simulink model "EMplanner_cs2018a"  (R2018a)
settings: Solver=ode5  StartTime=0.0  StopTime=50  FixedStep=1/1000  RelTol=1e-3
PreLoadFcn:
  | mbxruntime.callbacks.PreLoadFcn(bdroot);
PostLoadFcn:
  | mbxruntime.callbacks.PostLoadFcn(bdroot);
InitFcn:
  | mbxruntime.callbacks.InitFcn(bdroot);
StartFcn:
  | mbxruntime.callbacks.StartFcn(bdroot);
StopFcn:
  | mbxruntime.callbacks.StopFcn(bdroot);
model workspace (MAT data in the model file):
  mbox_table : struct (value not decoded)
  model_closed = 0
  sim_status = 0
values from neighbouring files (symbols this model uses):
  c_factor = 43.75    [emplanner_init.m]
  cf = -175016    [emplanner_init.m]
  cr = -130634    [emplanner_init.m]
  global_path_x = [-2.9245 -1.92511774493 -0.926994634419 0.0698522493473 1.06541712279 2.05969835808 3.05269585569 4.04441007764 5.03484169183 6.02399144113 7.01186009523 7.99844843293 ... (1201 elements, 1201x1)]    [global_path.mat]
  global_path_y = [13.2143 13.2143 13.2143 13.2143 13.2143 13.2143 13.2143 13.2143 13.2143 13.2143 13.2143 13.2143 ... (1201 elements, 1201x1)]    [global_path.mat]
  KD_PID_distance = 0.0    (= 0)    [emplanner_init.m]
  KD_PID_speed = 0    [emplanner_init.m]
  KI_PID_distance = 0.0    (= 0)    [emplanner_init.m]
  KI_PID_speed = 0    [emplanner_init.m]
  KP_PID_distance = 0.5    [emplanner_init.m]
  KP_PID_speed = 1.8    [emplanner_init.m]
  la = 1.265    [emplanner_init.m]
  lb = 2.947-1.265    (= 1.682)    [emplanner_init.m]
  LQR_K1 = k(:,1)'    [emplanner_init.m]
  LQR_K2 = k(:,2)'    [emplanner_init.m]
  LQR_K3 = k(:,3)'    [emplanner_init.m]
  LQR_K4 = k(:,4)'    [emplanner_init.m]
  m = 2020    [emplanner_init.m]
  rack_displacement = [-39.14 , -37.2 , -35.29 , -33.43 , -31.6 , -29.81 , -28.06 , -26.34 , -24.66 ,      -23.01 , -21.38 , -19.79 , -18.23 , -16.69 , -15.18 , -13.7 , -12.23 , -10.8 , -9.38 , -7.98 ,     -6.61 , -5.25 , -3.91 , -2.59 , -1.29 , 0 , 1.27 , 2.54 , 3.78 , 5.02 , 6.24 , 7.46 , 8.66 ,      9.86 , 11.05 , 12.24 , 13.41 , 14.59 , 15.76 , 16.92 , 18.09 , 19.25 , 20.42 , 21.59 , 22.76 ,      23.93 , 25.11 , 26 ...(+26 chars)    [emplanner_init.m]
  right_wheel_ground = [-70 ,-67.2 , -64.4 , -61.6 , -58.8 , -56 , -53.2 , -50.4 , -47.6 , -44.8 , -42 ,      -39.2 , -36.4 , -33.6 , -30.8 , -28 , -25.2 , -22.4 , -19.6 , -16.8 , -14 , -11.2 , -8.4 , -5.6 ,      -2.8 , 0 , 2.8 , 5.6 , 8.4 , 11.2 , 14 , 16.8 , 19.6 , 22.4 , 25.2 , 28 , 30.8 , 33.6 , 36.4 ,      39.2 , 42 , 44.8 , 47.6 , 50.4 , 53.2 , 56 , 58.8 , 61.6 , 64.4 , 67.2 , 70 ]    [emplanner_init.m]
  vx_break_point = zeros(1,5000)    [emplanner_init.m]
undefined symbols (not defined in the file or in its folder): aubr, DiscIntNeverNeededParam, tablebr, vubr, warningInitialVelocity, x0
libraries: simulink x19, simulink_extras x5, PreScanSimulinkLibrary x4, Solver_SF x1
(part 5 of 5)

== matlab function EMplanner_cs2018a/Audi_A8_Sedan_1/decision&planning module/referenceline provider/general fast algorithm to find projection point info ==
  data: x_set input; match_point_index_set output; y_set input; path_x input; path_y input; proj_x_set output; proj_y_set output; proj_heading_set output; proj_kappa_set output; path_heading input; path_kappa input
function [match_point_index_set,proj_x_set,proj_y_set,proj_heading_set,proj_kappa_set] = fcn(x_set,y_set,path_x,path_y,path_heading,path_kappa)
%该函数是一个通用函数，找到x_set,y_set在path_x,path_y的匹配点的编号，以及投影点在直角坐标系下的(x,y,theta,kappa)
%最多可以处理128个点

match_point_index_set = ones(128,1)*nan;
proj_x_set = ones(128,1)*nan;
proj_y_set = ones(128,1)*nan;
proj_heading_set = ones(128,1)*nan;
proj_kappa_set = ones(128,1)*nan;


persistent is_first_run;
persistent init_search_index_set;
if isempty(is_first_run)
    is_first_run = 0; 
    init_search_index_set = ones(128,1)*nan;
    for i = 1:length(x_set)
        if isnan(x_set(i))
            break;
        else
            increase_count = 0;
            min_distance = 1e10;
            for j = 1:length(path_x)
                distance = (x_set(i)-path_x(j))^2 + (y_set(i)-path_y(j))^2;
                if (min_distance > distance)
                    min_distance = distance;
                    init_search_index_set(i)=j;
                    increase_count = 0;
                else
                    increase_count = increase_count + 1;
                end
                if increase_count > 50
                    break;
                end
            end
            match_point_index = init_search_index_set(i);
            match_point_index_set(i) = match_point_index;
            vector_match_point = [path_x(match_point_index);path_y(match_point_index)];
            vector_match_point_direction = [cos(path_heading(match_point_index));sin(path_heading(match_point_index))];
            vector_host_point = [x_set(i);y_set(i)];
            vector_d = vector_host_point - vector_match_point;
            vector_err = (vector_d'* vector_match_point_direction) * vector_match_point_direction;
            vector_proj = vector_err + vector_match_point;
            proj_x_set(i) = vector_proj(1);
            proj_y_set(i) = vector_proj(2);
            proj_heading_set(i) = path_heading(match_point_index) + path_kappa(match_point_index) * (vector_d'* vector_match_point_direction);
            proj_kappa_set(i) = path_kappa(match_point_index);            
        end
    end 
else
    min_distance = inf;
    for i = 1:length(x_set)
        if isnan(x_set(i))
            break;
        else
            increase_count = 0;
            start_index = init_search_index_set(i);
            vector_m_init = [path_x(start_index);path_y(start_index)];
            vector_direction_init = [cos(path_heading(start_index));sin(path_heading(start_index))];
            ds = ([x_set(1);y_set(1)]-vector_m_init)'*vector_direction_init;
            if ds > 0            
                for j = start_index:length(path_x)
                    distance = (x_set(i)-path_x(j))^2 + (y_set(i)-path_y(j))^2;
                    if (min_distance > distance)
                        min_distance = distance;
                        init_search_index_set(i)=j;
                        increase_count = 0;
                    else
                        increase_count = increase_count + 1;
                    end
                    if increase_count > 3
                        break;
                    end
                end
            else
                for j = start_index:-1:1
                    distance = (x_set(i)-path_x(j))^2 + (y_set(i)-path_y(j))^2;
                    if (min_distance > distance)
                        min_distance = distance;
                        init_search_index_set(i)=j;
                        increase_count = 0;
                    else
                        increase_count = increase_count + 1;
                    end
                    if increase_count > 3
                        break;
                    end
                end
            end
            match_point_index = init_search_index_set(i);
            match_point_index_set(i) = match_point_index;
            vector_match_point = [path_x(match_point_index);path_y(match_point_index)];
            vector_match_point_direction = [cos(path_heading(match_point_index));sin(path_heading(match_point_index))];
            vector_host_point = [x_set(i);y_set(i)];
            vector_d = vector_host_point - vector_match_point;
            vector_err = (vector_d'* vector_match_point_direction) * vector_match_point_direction;
            vector_proj = vector_err + vector_match_point;
            proj_x_set(i) = vector_proj(1);
            proj_y_set(i) = vector_proj(2);
            proj_heading_set(i) = path_heading(match_point_index) + path_kappa(match_point_index) * (vector_d'* vector_match_point_direction);
            proj_kappa_set(i) = path_kappa(match_point_index);            
        end
    end    
end

== matlab function EMplanner_cs2018a/Audi_A8_Sedan_2/PathFollower_Preview_1/LateralController/Calculate delta steering error/eml_delta_steering_error ==
  data: v_x_vehicle input; v_x_vehicle_Min input; t_Preview_LatCtrl input; delta_steeringwheeltotal output; v_y_vehicle input; yawrate_vehicle input; CorneringStiffness_Tyres_Front input; CorneringStiffness_Tyres_Rear input; m_vehicle_total input; inertia_z_vehicle_total input; e_Lat input size=10; Pos_x_CoG_Vehicle input; wheelbase input; RefreshCounter parameter
function delta_steeringwheeltotal = eml_delta_steering_error(v_x_vehicle,v_x_vehicle_Min,t_Preview_LatCtrl,v_y_vehicle,yawrate_vehicle,CorneringStiffness_Tyres_Front,CorneringStiffness_Tyres_Rear,m_vehicle_total,inertia_z_vehicle_total,e_Lat,Pos_x_CoG_Vehicle,wheelbase,RefreshCounter)

delta_steeringwheeltotal = emlfcn_delta_steering_error(v_x_vehicle,v_x_vehicle_Min,t_Preview_LatCtrl,v_y_vehicle,yawrate_vehicle,CorneringStiffness_Tyres_Front,CorneringStiffness_Tyres_Rear,m_vehicle_total,inertia_z_vehicle_total,e_Lat,Pos_x_CoG_Vehicle,wheelbase,RefreshCounter);

% end function

== matlab function EMplanner_cs2018a/Audi_A8_Sedan_1/decision&planning module/referenceline provider/generate referenceline from global path ==
  data: global_path_x input; referenceline_x_init output; global_path_y input; host_match_point_index input; referenceline_y_init output
function [referenceline_x_init,referenceline_y_init] = fcn(global_path_x,global_path_y,host_match_point_index)
% 在host_match_point_index往前取150个点，往后取30个点，一共181个点
% 如果后面不够的话，比如后面只有5个点，那就后面取5个，前面取175个
% 如果前面点不够的话，同理往后面补，保证一共181个点

%索引初始化
start_index = -1;
end_index = -1;
host_index = host_match_point_index(1);
if host_index - 30 < 1 %判断后面的点是否足够
    start_index = 1;
    end_index = 181;
elseif host_index + 150 > length(global_path_x) %判断前面的点是否足够
        end_index = length(global_path_x);
        start_index = end_index - 180;
else
        start_index = host_index -30;
        end_index = host_index + 150;
end

referenceline_x_init = global_path_x(start_index:start_index + 180);
referenceline_y_init = global_path_y(start_index:start_index + 180);

== matlab function EMplanner_cs2018a/Audi_A8_Sedan_1/decision&planning module/referenceline provider/referenceline fem smoother with path splicing ==
  data: referenceline_x_init input; referenceline_x output; referenceline_y_init input; referenceline_x_init_pre input; referenceline_y_init_pre input; w_ref_cost input; w_smooth_cost input; w_length_cost input; referenceline_x_lb input; referenceline_x_ub input; referenceline_y_lb input; referenceline_y_ub input; referenceline_y output
function [referenceline_x,referenceline_y] = fcn(referenceline_x_init,referenceline_y_init,referenceline_x_init_pre,referenceline_y_init_pre,w_ref_cost,w_smooth_cost,w_length_cost,referenceline_x_lb,referenceline_x_ub,referenceline_y_lb,referenceline_y_ub)
coder.extrinsic("quadprog");
n=181;
%cost function =  w1*((xi-xiref)^2 + (yi - yiref)^2) +  w2*((xi+1 + xi-1 - 2*xi)^2 + (yi+1 + yi-1 - 2*yi)^2) + w3*((xi+1-xi)^2 + (yi+1 -yi)^2);
persistent is_first_run;
persistent pre_result_x;
persistent pre_result_y;
if isempty(is_first_run)
    is_first_run = 0;
    A1=zeros(2*n-4,2*n);
    A2=zeros(2*n-2,2*n);
    f=zeros(n*2,1);
    lb=f;
    ub=f;
    for i=1:n
    f(2*i-1)=referenceline_x_init(i);
    f(2*i)=referenceline_y_init(i);
    lb(2*i-1)=referenceline_x_init(i)-referenceline_x_lb;
    lb(2*i)=referenceline_y_init(i)-referenceline_y_lb;
    ub(2*i-1)=referenceline_x_init(i)+referenceline_x_ub;
    ub(2*i)=referenceline_y_init(i)+referenceline_y_ub;
    end

    for i=1:2:2*n-5
    A1(i,i)=1;
    A1(i,i+2)=-2;
    A1(i,i+4)=1;
    A1(i+1,i+1)=1;
    A1(i+1,i+3)=-2;
    A1(i+1,i+5)=1; 
    end
    for i=1:2:2*n-3
    A2(i,i)=1;
    A2(i,i+2)=-1;    
    A2(i+1,i+1)=1;
    A2(i+1,i+3)=-1;  
    end
    A3=eye(2*n,2*n);
    H=w_smooth_cost*(A1'*A1)+w_length_cost*(A2'*A2)+w_ref_cost*A3;
    H=2*H;
    X0=f;
    f=2*w_ref_cost*f;

    X=quadprog(H,f,[],[],[],[],lb,ub,X0);
    x=zeros(n,1);
    y=zeros(n,1);

    for i=1:n
    x(i)=X(2*i-1);
    y(i)=X(2*i);
    end

    referenceline_x=x;
    referenceline_y=y;
    
    pre_result_x = x;
    pre_result_y = y;
else
    %%%找到新的reference_line_init的起点在旧的referenceline的位置编号
    %编号初始化
    index = -1;
    new_init_point_x = referenceline_x_init(1);
    new_init_point_y = referenceline_y_init(1);
    for i = 1:length(referenceline_x_init_pre)
        if (new_init_point_x == referenceline_x_init_pre(i))&&(new_init_point_y == referenceline_y_init_pre(i))
            index = i;
            break;
        end
    end
    if (index == -1)||(index > 6)
        %没找到，或者超过6个，按照原来的方法处理
        A1=zeros(2*n-4,2*n);
        A2=zeros(2*n-2,2*n);
        f=zeros(n*2,1);
        lb=f;
        ub=f;
        for i=1:n
        f(2*i-1)=referenceline_x_init(i);
        f(2*i)=referenceline_y_init(i);
        lb(2*i-1)=referenceline_x_init(i)-referenceline_x_lb;
        lb(2*i)=referenceline_y_init(i)-referenceline_y_lb;
        ub(2*i-1)=referenceline_x_init(i)+referenceline_x_ub;
        ub(2*i)=referenceline_y_init(i)+referenceline_y_ub;
        end
        for i=1:2:2*n-5
        A1(i,i)=1;
        A1(i,i+2)=-2;
        A1(i,i+4)=1;
        A1(i+1,i+1)=1;
        A1(i+1,i+3)=-2;
        A1(i+1,i+5)=1; 
        end
        for i=1:2:2*n-3
        A2(i,i)=1;
        A2(i,i+2)=-1;    
        A2(i+1,i+1)=1;
        A2(i+1,i+3)=-1;  
        end
        A3=eye(2*n,2*n);
        H=w_smooth_cost*(A1'*A1)+w_length_cost*(A2'*A2)+w_ref_cost*A3;
        H=2*H;
        X0=f;
        f=2*w_ref_cost*f;

        X=quadprog(H,f,[],[],[],[],lb,ub,X0);
        x=zeros(n,1);
        y=zeros(n,1);

        for i=1:n
        x(i)=X(2*i-1);
        y(i)=X(2*i);
        end

        referenceline_x = x;
        referenceline_y = y;

        pre_result_x = x;
        pre_result_y = y;
    elseif index == 1
        %找到了，并且起点一摸一样
        referenceline_x = pre_result_x;
        referenceline_y = pre_result_y;
    else
        %找到了，但是起点不一样，但是还有一个问题，不知道到底需要拼接几个点，速度低的时候可能只需要去掉一个点，拼上一个点，但是速度高的时候可能需要去掉多个点在拼上多个点，优化矩阵是动态的
        %simulink不支持动态生成矩阵
        %解决方案是先申明一个最多处理6个点的优化矩阵，作为缓冲
        n1 = 6 + 2;%因为要带上原优化方案的最后两个点，所以最终的n = 6+2;
        A1=zeros(2*n1-4,2*n1);
        A2=zeros(2*n1-2,2*n1);
        f=zeros(n1*2,1);
        lb=f;
        ub=f;
        point_count = index - 1;%拼接点的数量
        
        f(1) = pre_result_x(length(referenceline_x_init) - 1);
        f(2) = pre_result_y(length(referenceline_x_init) - 1);
        f(3) = pre_result_x(length(referenceline_x_init));
        f(4) = pre_result_y(length(referenceline_x_init));
        lb(1) = f(1);
        ub(1) = f(1);
        lb(2) = f(2);
        ub(2) = f(2);
        lb(3) = f(3);
        ub(3) = f(3);
        lb(4) = f(4);
        ub(4) = f(4);
        
        start_index = length(referenceline_x_init) - point_count;
        for i=1:point_count
            f(2*(i+2)-1)=referenceline_x_init(start_index + i);
            f(2*(i+2))=referenceline_y_init(start_index + i);
            lb(2*(i+2)-1)=referenceline_x_init(start_index + i)-referenceline_x_lb;
            lb(2*(i+2))=referenceline_y_init(start_index + i )-referenceline_y_lb;
            ub(2*(i+2)-1)=referenceline_x_init(start_index + i)+referenceline_x_ub;
            ub(2*(i+2))=referenceline_y_init(start_index + i)+referenceline_y_ub;
        end
        for i=1:2:2*(point_count + 2) - 5
        A1(i,i)=1;
        A1(i,i+2)=-2;
        A1(i,i+4)=1;
        A1(i+1,i+1)=1;
        A1(i+1,i+3)=-2;
        A1(i+1,i+5)=1; 
        end
        for i=1:2:2*(point_count + 2) - 3
            A2(i,i)=1;
            A2(i,i+2)=-1;    
            A2(i+1,i+1)=1;
            A2(i+1,i+3)=-1;  
        end
        A3=eye(2*n1,2*n1);
        H=w_smooth_cost*(A1'*A1)+w_length_cost*(A2'*A2)+w_ref_cost*A3;
        H=2*H;
        X0=f;
        f=2*w_ref_cost*f;
        %二次规划
        X=quadprog(H,f,[],[],[],[],lb,ub,X0);
        x=zeros(point_count,1);
        y=zeros(point_count,1);

        for i=1:point_count
            x(i) = X(2*i + 3);
            y(i) = X(2*i + 4);
        end
        referenceline_x = zeros(n,1);
        referenceline_y = zeros(n,1);
        %轨迹拼接
        for i = 1:length(referenceline_x_init) 
            if i <= length(referenceline_x_init) - point_count
                referenceline_x(i) = pre_result_x(i + point_count);
                referenceline_y(i) = pre_result_y(i + point_count);
            else
                referenceline_x(i) = x(i - (length(referenceline_x_init) - point_count));
                referenceline_y(i) = y(i - (length(referenceline_y_init) - point_count));
            end
        end

  

        pre_result_x = referenceline_x;
        pre_result_y = referenceline_y;
  
        
        
        
    end
    
    
end

== matlab function EMplanner_cs2018a/Audi_A8_Sedan_1/decision&planning module/general fast algorithm to find projection point info ==
  data: x_set input; match_point_index_set output; y_set input; path_x input; path_y input; proj_x_set output; proj_y_set output; proj_heading_set output; proj_kappa_set output; path_heading input; path_kappa input
function [match_point_index_set,proj_x_set,proj_y_set,proj_heading_set,proj_kappa_set] = fcn(x_set,y_set,path_x,path_y,path_heading,path_kappa)
%该函数是一个通用函数，找到x_set,y_set在path_x,path_y的匹配点的编号，以及投影点在直角坐标系下的(x,y,theta,kappa)
%最多可以处理128个点

match_point_index_set = ones(128,1)*nan;
proj_x_set = ones(128,1)*nan;
proj_y_set = ones(128,1)*nan;
proj_heading_set = ones(128,1)*nan;
proj_kappa_set = ones(128,1)*nan;


persistent is_first_run;
persistent init_search_index_set;
if isempty(is_first_run)
    is_first_run = 0; 
    init_search_index_set = ones(128,1)*nan;
    for i = 1:length(x_set)
        if isnan(x_set(i))
            break;
        else
            increase_count = 0;
            min_distance = 1e10;
            for j = 1:length(path_x)
                distance = (x_set(i)-path_x(j))^2 + (y_set(i)-path_y(j))^2;
                if (min_distance > distance)
                    min_distance = distance;
                    init_search_index_set(i)=j;
                    increase_count = 0;
                else
                    increase_count = increase_count + 1;
                end
                if increase_count > 50
                    break;
                end
            end
            match_point_index = init_search_index_set(i);
            match_point_index_set(i) = match_point_index;
            vector_match_point = [path_x(match_point_index);path_y(match_point_index)];
            vector_match_point_direction = [cos(path_heading(match_point_index));sin(path_heading(match_point_index))];
            vector_host_point = [x_set(i);y_set(i)];
            vector_d = vector_host_point - vector_match_point;
            vector_err = (vector_d'* vector_match_point_direction) * vector_match_point_direction;
            vector_proj = vector_err + vector_match_point;
            proj_x_set(i) = vector_proj(1);
            proj_y_set(i) = vector_proj(2);
            proj_heading_set(i) = path_heading(match_point_index) + path_kappa(match_point_index) * (vector_d'* vector_match_point_direction);
            proj_kappa_set(i) = path_kappa(match_point_index);            
        end
    end 
else
    min_distance = inf;
    for i = 1:length(x_set)
        if isnan(x_set(i))
            break;
        else
            increase_count = 0;
            start_index = init_search_index_set(i);
            vector_m_init = [path_x(start_index);path_y(start_index)];
            vector_direction_init = [cos(path_heading(start_index));sin(path_heading(start_index))];
            ds = vector_m_init'*vector_direction_init;
            if ds > 0            
                for j = start_index:length(path_x)
                    distance = (x_set(i)-path_x(j))^2 + (y_set(i)-path_y(j))^2;
                    if (min_distance > distance)
                        min_distance = distance;
                        init_search_index_set(i)=j;
                        increase_count = 0;
                    else
                        increase_count = increase_count + 1;
                    end
                    if increase_count > 3
                        break;
                    end
                end
            else
                for j = start_index:-1:1
                    distance = (x_set(i)-path_x(j))^2 + (y_set(i)-path_y(j))^2;
                    if (min_distance > distance)
                        min_distance = distance;
                        init_search_index_set(i)=j;
                        increase_count = 0;
                    else
                        increase_count = increase_count + 1;
                    end
                    if increase_count > 3
                        break;
                    end
                end
            end
            match_point_index = init_search_index_set(i);
            match_point_index_set(i) = match_point_index;
            vector_match_point = [path_x(match_point_index);path_y(match_point_index)];
            vector_match_point_direction = [cos(path_heading(match_point_index));sin(path_heading(match_point_index))];
            vector_host_point = [x_set(i);y_set(i)];
            vector_d = vector_host_point - vector_match_point;
            vector_err = (vector_d'* vector_match_point_direction) * vector_match_point_direction;
            vector_proj = vector_err + vector_match_point;
            proj_x_set(i) = vector_proj(1);
            proj_y_set(i) = vector_proj(2);
            proj_heading_set(i) = path_heading(match_point_index) + path_kappa(match_point_index) * (vector_d'* vector_match_point_direction);
            proj_kappa_set(i) = path_kappa(match_point_index);            
        end
    end    
end

== matlab function EMplanner_cs2018a/Audi_A8_Sedan_1/decision&planning module/referenceline provider/calc path heading and kappa2(please do not use) ==
  data: path_x input; path_heading output; path_y input; path_kappa output
function [path_heading,path_kappa] = fcn(path_x,path_y)
dy = diff(path_y);
dx = diff(path_x);
path_theta_init1 = atan2(dy,dx);
% for i=1:length(path_theta_init1)
%     if path_theta_init1(i)<0
%        path_theta_init1(i) =  path_theta_init1(i) + pi;
%     end
% end
path_heading = [path_theta_init1;path_theta_init1(end)];


path_ds = sqrt(diff(path_y).^2+diff(path_x).^2);
path_dheading = sin(diff(path_heading));
path_kappa1 = path_dheading./path_ds;
path_kappa = [path_kappa1;path_kappa1(end)];

== matlab function EMplanner_cs2018a/Audi_A8_Sedan_1/control module/control main/longitudinal control double PID/MATLAB Function3 ==
  data: kp input; pid_out output; ki input; kd input; err input; err_delay input
function pid_out = fcn(kp,ki,kd,err,err_delay)

persistent integral;
if isempty(integral)
    integral = err * ki *0.01;
    devia = kd*(err - err_delay)/0.01;
    pid_out = kp*err + integral + devia;
else
    integral = integral + err * ki *0.01;
    devia = kd*(err - err_delay)/0.01;
    pid_out = kp*err + integral + devia;
end

== matlab function EMplanner_cs2018a/Audi_A8_Sedan_1/control module/control main/lateral control LQR/err_kappa_calculate_module ==
  data: x input; y input; phi input; vx input; vy input; phi_dot input; xr input; yr input; thetar input; kappar input; err output; es output; s_dot output
function [err,es,s_dot] = fcn(x,y,phi,vx,vy,phi_dot,xr,yr,thetar,kappar)
    
    tor=[cos(thetar);sin(thetar)];
    nor=[-sin(thetar);cos(thetar)];
    d_err=[x-xr;y-yr];
    ed=nor'*d_err;
    es=tor'*d_err;
    %projection_point_thetar=thetar(dmin);%apollo
    projection_point_thetar=thetar+kappar*es;
    ed_dot=vy*cos(phi-projection_point_thetar)+vx*sin(phi-projection_point_thetar);
    %%%%%%%%%
    ephi=sin(phi-projection_point_thetar);
    %%%%%%%%%
    ss_dot=vx*cos(phi-projection_point_thetar)-vy*sin(phi-projection_point_thetar);
    s_dot=ss_dot/(1-kappar*ed);
    ephi_dot=phi_dot-kappar*s_dot;
    err=[ed;ed_dot;ephi;ephi_dot];
    
    
    
    
    
    
    
    
    
    
    
    


end

== matlab function EMplanner_cs2018a/Audi_A8_Sedan_1/control module/control main/lateral control LQR/feed_forword_control ==
  data: vx input; a input; forword_angle output; b input; m input; cf input; cr input; k input; kr input
function forword_angle = fcn(vx,a,b,m,cf,cr,k,kr)
    forword_angle=kr*(a+b-b*k(3)-(m*vx*vx/(a+b))*((b/cf)+(a/cr)*k(3)-(a/cr)));
end

== matlab function EMplanner_cs2018a/Audi_A8_Sedan_1/control module/control main/lateral control LQR/feedback_control+feedforword_control ==
  data: k input; angle output; err input; forword_angle input
function angle = fcn(k,err,forword_angle)

    angle=-k*err+forword_angle;
end

== matlab function EMplanner_cs2018a/Audi_A8_Sedan_1/control module/control main/lateral control LQR/calc lqr K ==
  data: k1 input; k output; k2 input; k3 input; k4 input; vx input
function k  = fcn(k1,k2,k3,k4,vx)
    if abs(vx)<0.1
        k=[0,0,0,0];
    else
       
        k=[k1,k2,k3,k4];
    end
end

== matlab function EMplanner_cs2018a/Audi_A8_Sedan_1/control module/control main/lateral control LQR/predict_module ==
  data: x input; pred_x_ctrl output; y input; phi input; vx input; vy input; phi_dot input; ts input; pred_y_ctrl output; pred_yaw_ctrl output; pred_vx_ctrl output; pred_vy_ctrl output; pred_yaw_dot_ctrl output
function [pred_x_ctrl,pred_y_ctrl,pred_yaw_ctrl,pred_vx_ctrl,pred_vy_ctrl,pred_yaw_dot_ctrl] = fcn(x,y,phi,vx,vy,phi_dot,ts)
    pred_x_ctrl=x+vx*ts*cos(phi)-vy*ts*sin(phi);
    pred_y_ctrl=y+vy*ts*cos(phi)+vx*ts*sin(phi);
    pred_yaw_ctrl=phi;
    pred_vx_ctrl=vx;
    pred_vy_ctrl=vy;
    pred_yaw_dot_ctrl=phi_dot;
end
